simulink model "Prob_5"  (R2020b)
settings: Solver=VariableStepAuto  StartTime=0.0  StopTime=10.0  RelTol=1e-3
undefined symbols (not defined in the file): C, R
settings Model: Creator=kshir  LastModifiedBy=kshir

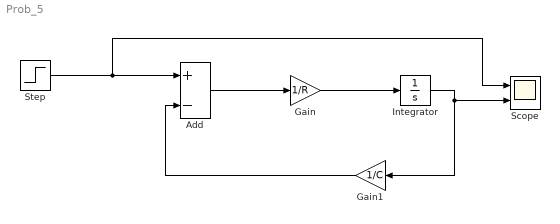
== system Prob_5 ==
  Add : Sum  Inputs=+-
  Gain : Gain  Gain=1/R
  Gain1 : Gain  Gain=1/C
  Integrator : Integrator
  Scope : Scope  NumInputPorts=2
  Step : Step  Time=2  After=4  SampleTime=0
  wires:
  Integrator/1 -> Scope/2, Gain1/1
  Gain/1 -> Integrator/1
  Gain1/1 -> Add/2
  Add/1 -> Gain/1
  Step/1 -> Add/1, Scope/1
